simulink model "PIDControllerRference"  (R2020b)
settings: Solver=VariableStepAuto  StartTime=0.0  StopTime=10.0  RelTol=1e-3
undefined symbols (not defined in the file): ki, kp, Ts
settings Model: Creator=lenovo  LastModifiedBy=lenovo

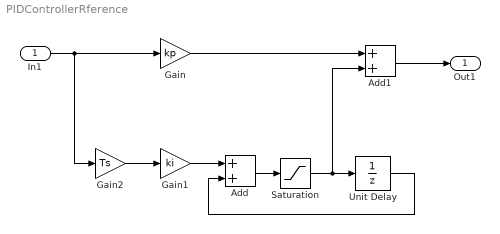
== system PIDControllerRference ==
  In1 : Inport
  Add : Sum
  Add1 : Sum
  Gain : Gain  Gain=kp
  Gain1 : Gain  Gain=ki
  Gain2 : Gain  Gain=Ts
  Saturation : Saturate
  Unit Delay : UnitDelay  SampleTime=-1  HasFrameUpgradeWarning=on
  Out1 : Outport
  wires:
  In1/1 -> Gain2/1, Gain/1
  Gain1/1 -> Add/1
  Gain2/1 -> Gain1/1
  Add/1 -> Saturation/1
  Unit Delay/1 -> Add/2
  Saturation/1 -> Add1/2, Unit Delay/1
  Gain/1 -> Add1/1
  Add1/1 -> Out1/1
